simulink model "ACKERMANN_MODEL"  (R2023b)
settings: Solver=VariableStepAuto  StartTime=0.0  StopTime=inf  RelTol=1e-3
undefined symbols (not defined in the file): DWORK0, DWORK1, initState, kd, ki, kp, maximumSteeringAngle, noisePower, sampleNoiseTime, sampleTimePID, slewRateNeg, slewRatePos, waypoints
libraries: simulink x3, robotmobilelib x1, slpidlib x1
settings Model: SILPILSystemUnderTest=refmodels  Creator=pabloafonsoyanes  LastModifiedBy=pabloafonsoyanes
settings OptimizationCC: DefaultParameterBehavior=Inlined  EnhancedBackFolding=on  PassReuseOutputArgsAs=Individual arguments  ZeroExternalMemoryAtStartup=off  ZeroInternalMemoryAtStartup=off  OptimizeBlockOrder=speed  DifferentSizesBufferReuse=on  OptimizationCustomize=off  EfficientTunableParamExpr=on
settings DebuggingCC: ParameterTunabilityLossMsg=error
settings HardwareCC: ProdBitPerLong=64  ProdHWDeviceType=Intel->x86-64 (Mac OS X)
settings SFSimCC: MATLABDynamicMemAlloc=off
settings RTWCC: Description=Embedded Coder  SystemTargetFile=ert.tlc  TemplateMakefile=ert_default_tmf
settings CodeAppCC: ForceParamTrailComments=on  IgnoreCustomStorageClasses=off  OperatorAnnotations=on  SimulinkDataObjDesc=on  SFDataObjDesc=on  InsertBlockDesc=on
settings ERTTargetCC: TargetLangStandard=C99 (ISO)  GenerateSampleERTMain=on  InlinedParameterPlacement=NonHierarchical  ERTCustomFileTemplate=example_file_process.tlc

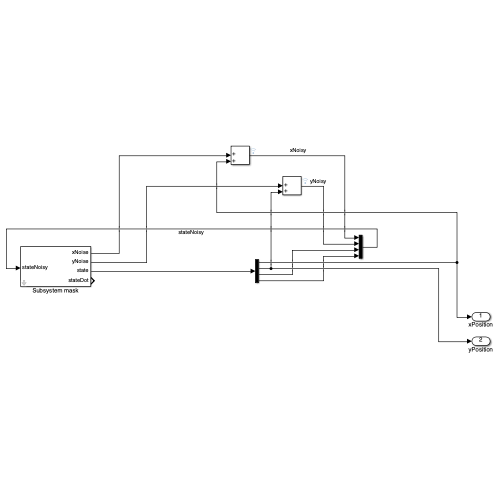
[thumbnail: Simulink's stored preview of the top-level diagram]
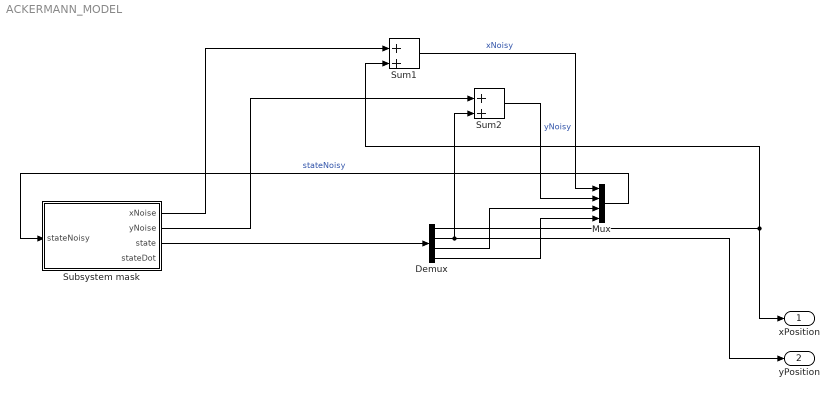
== system ACKERMANN_MODEL ==
  Demux : Demux
  Mux : Mux
  Subsystem mask : Subsystem  mask{waypoints=waypoints, slewRatePos=slewRatePos, slewRateNeg=slewRateNeg, sampleNoiseTime=sampleNoiseTime, maximumSteeringAngle=maximumSteeringAngle, noisePower=noisePower, kp=kp, ki=ki, kd=kd, initState=initState, sampleTimePID=sampleTimePID}
      mask prompts: waypoints "Waypoints (2xN matrix)"; slewRatePos "Positive Slew Rate"; slewRateNeg "Negative Slew Rate"; sampleNoiseTime "Sample Time for White Noise"; maximumSteeringAngle "Maximum Steering Angle"; noisePower "Noise Power for White Noise"; kp "Proportional Gain (kp)"; ki "Integral Gain (ki)"; kd "Derivative Gain (kd)"; initState "Initial State of Ackermann Kinematic Model"; sampleTimePID "Sample Time for PID Controller"
  Sum1 : Sum  Inputs=|++
  Sum2 : Sum  Inputs=|++
  xPosition : Outport
  yPosition : Outport  Port=2
  wires:
  Demux/1 -> xPosition/1, Sum1/2
  Demux/2 -> yPosition/1, Sum2/2
  Demux/3 -> Mux/3
  Sum2/1 -> Mux/2  "yNoisy"
  Sum1/1 -> Mux/1  "xNoisy"
  Demux/4 -> Mux/4
  Mux/1 -> Subsystem mask/1(stateNoisy)  "stateNoisy"
  Subsystem mask/1(xNoise) -> Sum1/1
  Subsystem mask/2(yNoise) -> Sum2/1
  Subsystem mask/3(state) -> Demux/1

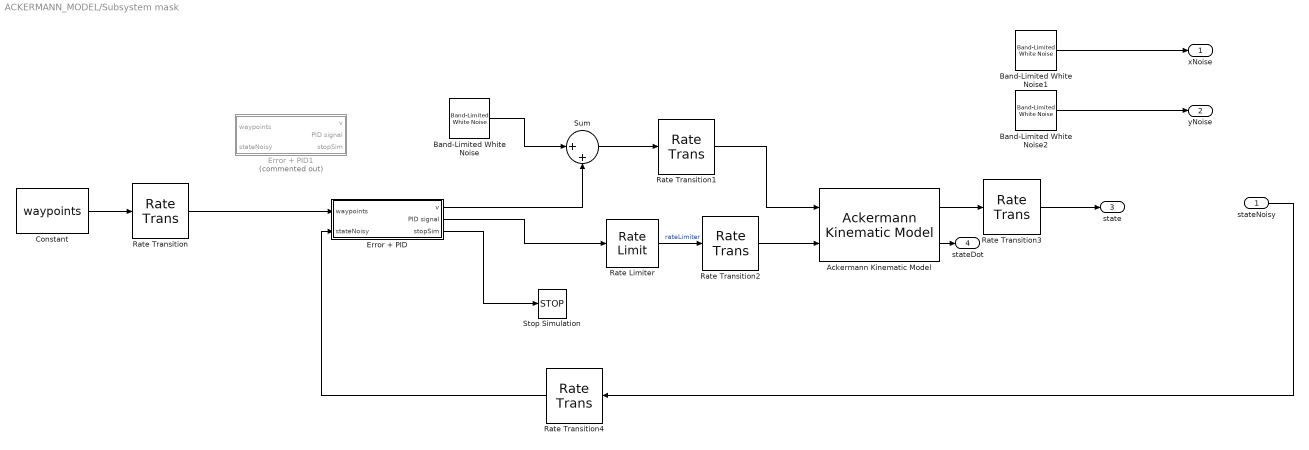
== system ACKERMANN_MODEL/Subsystem mask ==
  stateNoisy : Inport
  Ackermann Kinematic Model : robotmobilelib/Ackermann Kinematic Model  WheelBase=1  VehicleSpeedRange=[0 100]  MaxSteeringAngle=maximumSteeringAngle  InitialState=initState  SimulateUsing=Interpreted execution
  Band-Limited White Noise : simulink/Sources/Band-Limited White Noise  Cov=noisePower  Ts=sampleNoiseTime  seed=[23341]
  Band-Limited White Noise1 : simulink/Sources/Band-Limited White Noise  Cov=noisePower  Ts=sampleNoiseTime  seed=[23341]
  Band-Limited White Noise2 : simulink/Sources/Band-Limited White Noise  Cov=noisePower  Ts=sampleNoiseTime  seed=[23341]
  Constant : Constant  Value=waypoints
  Error + PID : Subsystem
  Error + PID1 : Subsystem  Commented=on
      mask help: Simulink:masks:GenSFuncDesc_MD
      mask Help: eval('feval(''rtwprivate'',''rtwhelpview'',''rtw_sfcn_block'')');
  Rate Limiter : RateLimiter  RisingSlewLimit=slewRatePos  FallingSlewLimit=slewRateNeg  SampleTimeMode=inherited
  Rate Transition{,2..4} (4 alike) : RateTransition  OutPortSampleTime=1/100
  Rate Transition1 : RateTransition  OutPortSampleTime=1/10
  Stop Simulation : Stop
  Sum : Sum  Inputs=|++
  xNoise : Outport
  yNoise : Outport  Port=2
  state : Outport  Port=3
  stateDot : Outport  Port=4
  wires:
  stateNoisy/1 -> Rate Transition4/1
  Band-Limited White Noise2/1 -> yNoise/1
  Constant/1 -> Rate Transition/1
  Rate Transition3/1 -> state/1
  Sum/1 -> Rate Transition1/1
  Band-Limited White Noise/1 -> Sum/1
  Rate Transition1/1 -> Ackermann Kinematic Model/1
  Rate Transition2/1 -> Ackermann Kinematic Model/2
  Ackermann Kinematic Model/1 -> Rate Transition3/1
  Band-Limited White Noise1/1 -> xNoise/1
  Ackermann Kinematic Model/2 -> stateDot/1
  Rate Limiter/1 -> Rate Transition2/1  "rateLimiter"
  Rate Transition/1 -> Error + PID/1(waypoints)
  Error + PID/1(v) -> Sum/2
  Error + PID/2(PID signal) -> Rate Limiter/1
  Error + PID/3(stopSim) -> Stop Simulation/1
  Rate Transition4/1 -> Error + PID/2(stateNoisy)

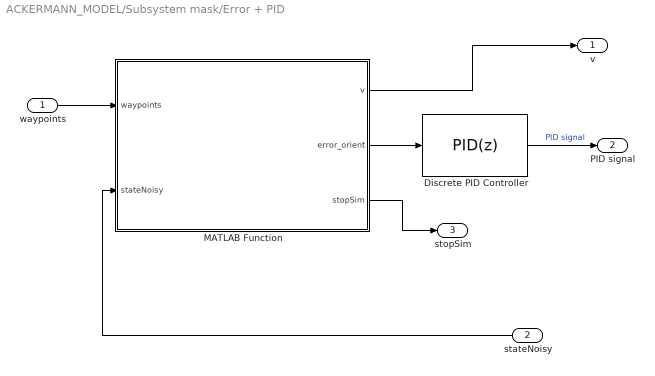
== system ACKERMANN_MODEL/Subsystem mask/Error + PID ==
  waypoints : Inport
  stateNoisy : Inport  Port=2
  Discrete PID Controller : slpidlib/PID Controller  Controller=PID  Form=Parallel  TimeDomain=Discrete-time  UseExternalTs=off  SampleTime=sampleTimePID  IntegratorMethod=Forward Euler  FilterMethod=Forward Euler  ControllerParametersSource=internal  P=kp  I=ki  UseKiTs=on  D=kd  N=100  UseFilter=on  TunerSelectOption=Transfer Function Based (PID Tuner App)  InitialConditionSource=internal  InitialConditionForIntegrator=0  InitialConditionForFilter=0  DifferentiatorICPrevScaledInput=0  ExternalReset=none  TrackingMode=off  Kt=1  LimitOutput=on  SatLimitsSource=internal  UpperSaturationLimit=pi/4  LowerSaturationLimit=-pi/4  LinearizeAsGain=off  AntiWindupMode=back-calculation  Kb=0.1  LimitIntegrator=off  UpperIntegratorSaturationLimit=inf  LowerIntegratorSaturationLimit=-inf  POutMin=[]  POutMax=[]  IOutMin=[]  IOutMax=[]  DOutMin=[]  DOutMax=[]  NOutMin=[]  NOutMax=[]  SumOutMin=[]  SumOutMax=[]  SaturationOutMin=[]  SaturationOutMax=[]  PParamMin=[]  PParamMax=[]  IParamMin=[]  IParamMax=[]  DParamMin=[]  DParamMax=[]  NParamMin=[]  NParamMax=[]  KbParamMin=[]  KbParamMax=[]  KtParamMin=[]  KtParamMax=[]  KbOutMin=[]  KbOutMax=[]  KtOutMin=[]  KtOutMax=[]  IntegratorOutMin=[]  IntegratorOutMax=[]  FilterOutMin=[]  FilterOutMax=[]  SumI1OutMin=[]  SumI1OutMax=[]  SumI2OutMin=[]  SumI2OutMax=[]  SumI3OutMin=[]  SumI3OutMax=[]  SumI4OutMin=[]  SumI4OutMax=[]  SumDOutMin=[]  SumDOutMax=[]  DifferentiatorOutMin=[]  DifferentiatorOutMax=[]  FilterDiffOutCoefMin=[]  FilterDiffOutCoefMax=[]  ReciprocalOutMin=[]  ReciprocalOutMax=[]  SumDenOutMin=[]  SumDenOutMax=[]  SumNumOutMin=[]  SumNumOutMax=[]  DivideOutMin=[]  DivideOutMax=[]  UdiffTsProdOutMin=[]  UdiffTsProdOutMax=[]  NTsProdOutMin=[]  NTsProdOutMax=[]  UintegralTsProdOutMin=[]  UintegralTsProdOutMax=[]  UngainTsProdOutMin=[]  UngainTsProdOutMax=[]  ClampingZeroOutDataTypeStr=Inherit: Inherit via back propagation  ClampingZeroOutMin=[]  ClampingZeroOutMax=[]  FilterDenConstantOutDataTypeStr=Inherit: Inherit via back propagation  FilterDenConstantOutMin=[]  FilterDenConstantOutMax=[]  PCopyOutDataTypeStr=Inherit: Inherit via back propagation  PCopyOutMin=[]  PCopyOutMax=[]  NCopyOutDataTypeStr=Inherit: Inherit via back propagation  NCopyOutMin=[]  NCopyOutMax=[]  IntegratorContinuousStateAttributes=''  IntegratorStateMustResolveToSignalObject=off  IntegratorRTWStateStorageClass=Auto  FilterContinuousStateAttributes=''  FilterStateMustResolveToSignalObject=off  FilterRTWStateStorageClass=Auto  ParallelPVariant=InternalParameters  IdealPVariant=Disabled  IVariant=InternalParameters  DVariant=InternalParameters  IntegratorVariant=Discrete  SatVariant=Enabled  AWVariant=BackCalculation  PCopyVariant=Disabled  TRVariant=Disabled  FdbkBlocksVariant=Forward  IdealPFdbkVariant=Disabled  SatFdbkVariant=Disabled  DerivativeFilterVariant=ForwardEulerFilter  NVariant=InternalParameters  NCopyVariant=Disabled  FilterICVariant=InternalICsFilter  IntegratorICVariant=InternalICs  ExternalResetVariant=Disabled  TRSumVariant=Passthrough  SumFdbkVariant=Disabled  SumVariant=Sum_PID  TsampFilterVariant=InternalTs  TsampNgainVariant=Passthrough  TsampIntegralVariant=Disabled_SignalSpec  ExternalSaturationOutDataTypeStr=Inherit: Same as second input
      settings: LibrarySourceBlock=simulink/Discrete/Discrete PID Controller
  MATLAB Function : MATLAB Function  TreatAsAtomicUnit=on
  v : Outport
  PID signal : Outport  Port=2
  stopSim : Outport  Port=3
  wires:
  MATLAB Function/1(v) -> v/1
  MATLAB Function/3(stopSim) -> stopSim/1
  waypoints/1 -> MATLAB Function/1(waypoints)
  Discrete PID Controller/1 -> PID signal/1  "PID signal"
  stateNoisy/1 -> MATLAB Function/2(stateNoisy)
  MATLAB Function/2(error_orient) -> Discrete PID Controller/1

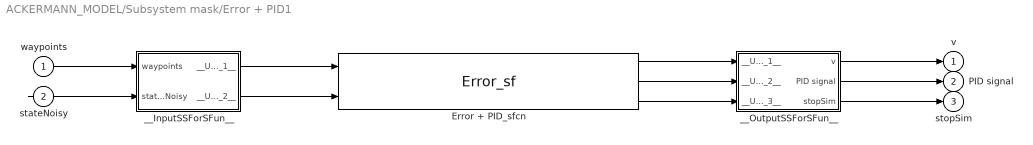
== system ACKERMANN_MODEL/Subsystem mask/Error + PID1 ==
  waypoints : Inport
  stateNoisy : Inport  Port=2
  Error + PID_sfcn : S-Function  FunctionName=Error_sf  SFunctionModules=""  SFunctionDeploymentMode=off  EnableBusSupport=off  SFcnStateName=DWORK0,DWORK1  mask{rtw_sf_name=Error_sf, showVar=off}
      mask prompts: rtw_sf_name "Simulink:masks:GenSFuncName_MP"; showVar "Simulink:masks:GenSFuncShowModuleList_MP"
      mask help: Simulink:masks:GenSFuncDesc_MD
      mask init:
      | displist = '';
      | if ~strcmp(get_param(gcb, 'FunctionName'), rtw_sf_name);
      |   set_param(gcb, 'FunctionName', rtw_sf_name);
      | end
      | % Check if we are generating code
      | rtw_mode = false;
      | if strcmpi(get_param(bdroot(gcb),'SimulationStatus'),'Initializing')
      | 	rtw_mode = strcmpi(get_param(bdroot(gcb),'BuildingRTWCode'),'on') && ...
      | 		~strcmpi(get_param(bdroot(gcb),'TargetStyle'),'SimulationTarget');
      | end
      | if showVar || rtw_mode
      | 	if exist('rtwsfunc') == 2 | exist('rtwsfunc') == 6
      | 		tmplist = rtwsfunc(rtw_sf_name,gcb);
      | 		tmplist = DAStudio.message('Simulink:masks:GenSFuncListOfModules_IC', tmplist);
      | 	elseif showVar
      | 		tmplist1 = DAStudio.message('Simulink:masks:GenSFuncListOfModules_IC', '');
      |         tmplist2 = DAStudio.message('Simulink:masks:GenSFuncNotLicensed_IC');
      |         tmplist = [tmplist1 tmplist2];
      |  	end
      | end
      | if showVar
      |   displist = tmplist;
      | end
      settings: SFcnIsStateOwnerBlock=on
      settings: CopyFcn=|
      | if ~strcmp(get_param(gcb,'Linkstatus'),'none') && ...
      | ~strcmp(get_param(gcb,'Linkstatus'),'implicit')
      |   set_param(gcb,'LinkStatus','none');
      | end
      mask Help: eval('feval(''rtwprivate'',''rtwhelpview'',''rtw_sfcn_block'')');
      mask Display:
      | port_label('input',1,'waypoints');
      | port_label('input',2,'stateNoisy');
      | port_label('output',1,'v');
      | port_label('output',2,'PID signal');
      | port_label('output',3,'stopSim');
  __InputSSForSFun__ : Subsystem
  __OutputSSForSFun__ : Subsystem
  v : Outport
  PID signal : Outport  Port=2
  stopSim : Outport  Port=3
  wires:
  waypoints/1 -> __InputSSForSFun__/1(waypoints)
  stateNoisy/1 -> __InputSSForSFun__/2(stateNoisy)
  __InputSSForSFun__/1(__UniqueOutportName__1__) -> Error + PID_sfcn/1
  __InputSSForSFun__/2(__UniqueOutportName__2__) -> Error + PID_sfcn/2
  Error + PID_sfcn/1 -> __OutputSSForSFun__/1(__UniqueInportName__1__)
  Error + PID_sfcn/2 -> __OutputSSForSFun__/2(__UniqueInportName__2__)
  Error + PID_sfcn/3 -> __OutputSSForSFun__/3(__UniqueInportName__3__)
  __OutputSSForSFun__/1(v) -> v/1
  __OutputSSForSFun__/2(PID signal) -> PID signal/1
  __OutputSSForSFun__/3(stopSim) -> stopSim/1

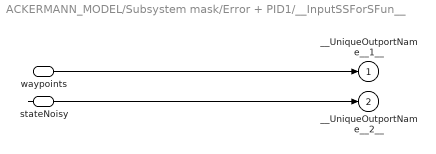
== system ACKERMANN_MODEL/Subsystem mask/Error + PID1/__InputSSForSFun__ ==
  waypoints : Inport
  stateNoisy : Inport  Port=2
  __UniqueOutportName__1__ : Outport
  __UniqueOutportName__2__ : Outport  Port=2
  wires:
  waypoints/1 -> __UniqueOutportName__1__/1
  stateNoisy/1 -> __UniqueOutportName__2__/1

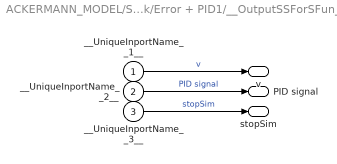
== system ACKERMANN_MODEL/Subsystem mask/Error + PID1/__OutputSSForSFun__ ==
  __UniqueInportName__1__ : Inport
  __UniqueInportName__2__ : Inport  Port=2
  __UniqueInportName__3__ : Inport  Port=3
  v : Outport
  PID signal : Outport  Port=2
  stopSim : Outport  Port=3
  wires:
  __UniqueInportName__1__/1 -> v/1  "v"
  __UniqueInportName__2__/1 -> PID signal/1  "PID signal"
  __UniqueInportName__3__/1 -> stopSim/1  "stopSim"

== matlab function ACKERMANN_MODEL/Subsystem mask/Error + PID/MATLAB Function ==
  data: v output; waypoints input; error_orient output; stateNoisy input; stopSim output
function [v, error_orient, stopSim] = calcOrientation(waypoints, stateNoisy)
    % calcOrientationErrorUnicycle: Calcula el error de orientación para 
    % un modelo unicycle/Ackermann simplificado que luego se controlará
    % mediante un PID discreto en Simulink (la salida del PID será la 
    % velocidad de giro w, aquí no la calculamos).
    %
    % Entradas:
    %   - waypoints: matriz 2xN con [x; y] de cada waypoint.
    %   - stateNoisy: [x, y, theta] (posición y orientación actual, con ruido).
    %
    % Salidas:
    %   - v: velocidad lineal (fija o variable, según prefieras).
    %   - error_orient: error de orientación (rango [-pi, pi]).
    %   - stopSim: bandera para detener la simulación (1 si se completaron todos los waypoints).

    % ========== 1) Variables persistentes: índice del waypoint ==========
    persistent idx
    if isempty(idx)
        idx = 1;  % Empezamos en el primer waypoint
    end

    % ========== 2) Parámetros y salidas por defecto ==========
    threshold = 0.25;  % Distancia mínima para dar por alcanzado un waypoint
    stopSim = 0;      % No detener la simulación por defecto
    v = 0.005;            % Velocidad lineal fija (ajusta según tu escenario)
    
    % ========== 3) Extraer el estado actual ==========
    x_actual = stateNoisy(1);
    y_actual = stateNoisy(2);
    theta_actual = stateNoisy(3);

    % ========== 4) Verificar si ya superamos el último waypoint ==========
    if idx > size(waypoints, 2)
        % Si ya no hay más waypoints
        stopSim = 1;         % Señal para detener la simulación
        v = 0;               % Opcional: pones velocidad a 0
        error_orient = 0;    % Sin error de orientación
        return;
    end

    % ========== 5) Waypoint actual ==========
    x_ref = waypoints(1, idx);
    y_ref = waypoints(2, idx);

    % ========== 6) Distancia al waypoint actual ==========
    dx = x_ref - x_actual;
    dy = y_ref - y_actual;
    dist = sqrt(dx^2 + dy^2);

    % ========== 7) Avanzar al siguiente waypoint si se alcanza el threshold ==========
    if dist < threshold
        if idx < size(waypoints, 2)
            idx = idx + 1;  % Pasar al siguiente waypoint
        else
            % Si era el último, detenemos
            stopSim = 1;
        end
    end

    % ========== 8) Cálculo del ángulo deseado y error de orientación ==========
    % Ángulo deseado para apuntar al waypoint actual
    angulo_deseado = atan2(dy, dx);

    % Error de orientación (ajustado a [-pi, pi])
    error_orient = angulo_deseado - theta_actual;
    error_orient = atan2(sin(error_orient), cos(error_orient));
end
